simulink model "generator"  (Simulink 3.00)
settings: Solver=ode4  StartTime=0.0  StopTime=100  FixedStep=0.1  RelTol=1e-3
settings Model: LastModifiedBy=Administrator

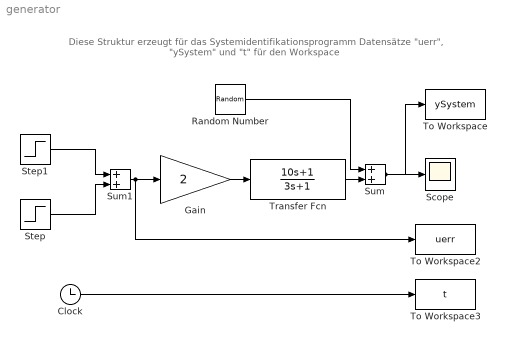
== system generator ==
  note: Diese Struktur erzeugt für das Systemidentifikationsprogramm
      | Datensätze "uerr", "ySystem" und "t" für den Workspace
  Clock : Clock
      settings: DisplayTime=off  Decimation=10
  Gain : Gain  Gain=2  SaturateOnIntegerOverflow=on
  Random Number : RandomNumber  Mean=0  Variance=0.005  Seed=0  SampleTime=0
  Scope : Scope
      settings: TimeRange=100  YMin=-450  YMax=50  SaveToWorkspace=off  SaveName=ScopeData  LimitMaxRows=off
  Step : Step  Time=50  Before=0  After=1  SampleTime=0
  Step1 : Step  Time=0  Before=0  After=1.5  SampleTime=0
  Sum : Sum  Inputs=++  SaturateOnIntegerOverflow=on
  Sum1 : Sum  Inputs=++  SaturateOnIntegerOverflow=on
  To Workspace : ToWorkspace  VariableName=ySystem  SampleTime=-1  SaveFormat=Matrix
  To Workspace2 : ToWorkspace  VariableName=uerr  SampleTime=-1  SaveFormat=Matrix
  To Workspace3 : ToWorkspace  VariableName=t  SampleTime=-1  SaveFormat=Matrix
  Transfer Fcn : TransferFcn  Numerator=[10 1]  Denominator=[3 1]
  wires:
  Transfer Fcn/1 -> Sum/2
  Step1/1 -> Sum1/1
  Step/1 -> Sum1/2
  Clock/1 -> To Workspace3/1
  Sum/1 -> Scope/1, To Workspace/1
  Gain/1 -> Transfer Fcn/1
  Sum1/1 -> To Workspace2/1, Gain/1
  Random Number/1 -> Sum/1
